simulink model "carTrailerModelDampened"  (R2018b)
settings: Solver=VariableStepAuto  StartTime=0.0  StopTime=StopTime  MaxStep=MaxStep  RelTol=1e-3
InitFcn:
  | SimFramework('model_parameters.json');
model workspace (MAT data in the model file):
  E = 0
  F = 5000
  MaxStep = 0.01
  StopTime = 475
  a1 = 5
  a2 = 2.5
  c = 0
  g = 9.8
  k = 12150
  m1 = 1400
  m2 = 600
  name = 'carTrailerModelDampened'
  u = 0.002
undefined symbols (not defined in the file or in its folder): magnitude
settings Model: Creator=rgeddes  LastModifiedBy=james

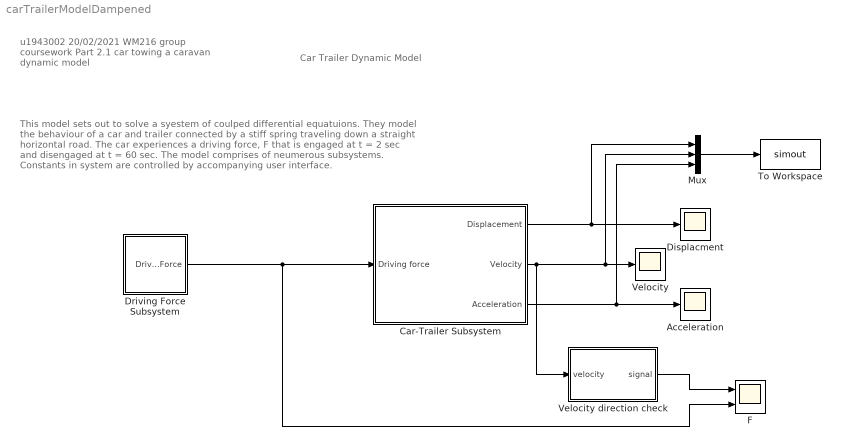
== system carTrailerModelDampened ==
  note: u1943002
      | 20/02/2021
      | WM216 group coursework
      | Part 2.1 car towing a caravan dynamic model
  note: This model sets out to solve a syestem of coulped differential equatuions.
      | They model the behaviour of a car and trailer connected by a stiff spring
      | traveling down a straight horizontal road. The car experiences a driving force, F
      | that is engaged at t = 2 sec and disengaged at t = 60 sec.
      | The model comprises of neumerous subsystems.
      | Constants in system are controlled by accompanying user interface.
  note: Car Trailer Dynamic Model
  Acceleration : Scope
  Car-Trailer Subsystem : Subsystem
      mask help: Combines the behaviour of two ordinary differential equations. Frictional and driving forces can be combined into separate equations for the car and trailer each. The spring force on each body is dependent on the relative displacement between the two bodies. A dampening system was introduced to reduce oscillations.
      mask init:
      | %default values
      | % m1 = 1400;
      | % m2 = 600;
      | % u = 0.002;
      | % a1 = 5;
      | % a2 = 2.5;
      | % g = 9.8;
      | % k = 3*(1800 + 250*9);
      | % c = 0
      | % E = 0
  Displacment : Scope
  Driving Force Subsystem : Subsystem
      mask help: Provindes the driving force F(t) as a function of time.
  F : Scope  NumInputPorts=2
  Mux : Mux  Inputs=3
  To Workspace : ToWorkspace  VariableName=simout  SampleTime=-1
  Velocity : Scope
  Velocity direction check : Subsystem
      mask help: Acts as a way of checking the length of simulation is sufficient. The end of the simulation is determined by visually approximating the point at which the velocity of either the car or trailer becomes negative. This is scaled to the magnitude of driving force, so they are comparable on the same scope.
      mask Help: The time at which peaks on the scoped output  begin reapear after the initial driving force stops can be taken as the time the simulation can be ended.
  wires:
  Car-Trailer Subsystem/3(Acceleration) -> Mux/3, Acceleration/1
  Car-Trailer Subsystem/2(Velocity) -> Velocity direction check/1(velocity), Mux/2, Velocity/1
  Car-Trailer Subsystem/1(Displacement) -> Mux/1, Displacment/1
  Mux/1 -> To Workspace/1
  Velocity direction check/1(signal) -> F/1
  Driving Force Subsystem/1(Driving Force) -> F/2, Car-Trailer Subsystem/1(Driving force)

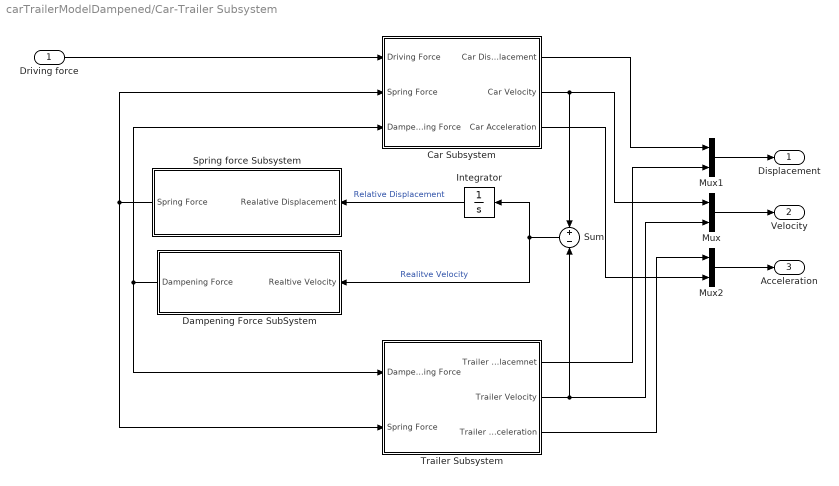
== system carTrailerModelDampened/Car-Trailer Subsystem ==
  Driving force : Inport
  " Car Subsystem" : Subsystem
      mask help:
      | The ODE modeling the behaviour of the car with dampening terms included.
      | x ̈_1=  (F(t))/m_1 -gμx ̇_1-a_1/m_1  〖x ̇_1〗^2-k/m_1  (x_1-x_2 )-c/m_1 (x ̇_1-x ̇_2)
      mask Help:
      | x ̈_1=  (F(t))/m_1 -gμx ̇_1-a_1/m_1  〖x ̇_1〗^2-k/m_1  (x_1-x_2 )-c/m_1 (x ̇_1-x ̇_2)
      | where
      | x _1 is the displacement of the car and its derivatives are given by dot notation.
      | F(t) is the driving force as a function of time.
      | m_1 is the mass of the car.
      | g is acceleration due to gravity.
      | μ is the coefficient of friction.
      | a_1 is the coefficient of air resistance for the car.
      | k is the spring force constant.
      | x_2 is the displacement of the trailer.
      | c is the dampening constant.
  Dampening Force SubSystem : Subsystem
      mask help: As the system undergoes oscilation a dampning sytem was included to explor its effectiveness in reducing oscilations. the dampening force is proportional to the relative velocity between the two bodies. F_d = c (x ̇_1-x ̇_2). the system contains an enable pin to allow the effects of dampening to be turned on and off.
      mask Help:
      | F_d = c (x ̇_1-x ̇_2)
      | where
      | F_d is the dampening force.
      | c is the dampening constant.
      | x ̇_1 is the velocity of the car.
      | x ̇_2 is the velocity of the trailer.
  Integrator : Integrator
  Mux : Mux  Inputs=2
  Mux1 : Mux  Inputs=2
  Mux2 : Mux  Inputs=2
  Spring force Subsystem : Subsystem
      mask help:
      | Spring force is proportional to the length of extension. Extension is given by the difference in displacement between the car and trailer.
      | F_s = k(x_1-x_2)
      mask Help:
      | F_s = k(x_1-x_2)
      | where
      | F_s is the spring force.
      | k is the spring constant.
      | x_1 is the displacement of the car.
      | x_2 is the displacemnet of the trailer.
  Sum : Sum  Inputs=+-
  Trailer Subsystem : Subsystem
      mask help:
      | The ODE modeling the behaviour of the trailer. With dampening terms included.
      | x ̈_2= -gμx ̇_2-a_2/m_2  〖x ̇_1〗^2+k/m_2  (x_1-x_2 )+c/m_2 (x ̇_1-x ̇_2)
      mask Help:
      | x ̈_2= -gμx ̇_2-a_2/m_2  〖x ̇_1〗^2+k/m_2  (x_1-x_2 )+c/m_2 (x ̇_1-x ̇_2)
      | where
      | x _2 is the displacement of the car and its derivatives are given by dot notation.
      | m_2 is the mass of the trailer.
      | g is acceleration due to gravity.
      | μ is the coefficient of friction.
      | a_2 is the coefficient of air resistance for the trailer.
      | k is the spring force constant.
      | x_1 is the displacement of the car.
      | c is the dampening constant.
  Displacement : Outport  VectorParamsAs1DForOutWhenUnconnected=off
  Velocity : Outport  Port=2  VectorParamsAs1DForOutWhenUnconnected=off
  Acceleration : Outport  Port=3  VectorParamsAs1DForOutWhenUnconnected=off
  wires:
  Mux2/1 -> Acceleration/1
  Driving force/1 -> " Car Subsystem"/1(Driving Force)
  Sum/1 -> Dampening Force SubSystem/1(Realtive Velocity), Integrator/1  "Realitve Velocity"
  Spring force Subsystem/1(Spring Force) -> Trailer Subsystem/2(Spring Force), " Car Subsystem"/2(Spring Force)
  Trailer Subsystem/1(Trailer Displacemnet) -> Mux1/2
  " Car Subsystem"/1(Car Displacement) -> Mux1/1
  Trailer Subsystem/3(Trailer Acceleration) -> Mux2/1
  " Car Subsystem"/3(Car Acceleration) -> Mux2/2
  " Car Subsystem"/2(Car Velocity) -> Sum/1, Mux/1
  Trailer Subsystem/2(Trailer Velocity) -> Mux/2, Sum/2
  Mux/1 -> Velocity/1
  Mux1/1 -> Displacement/1
  Integrator/1 -> Spring force Subsystem/1(Realative Displacement)  "Relative Displacement"
  Dampening Force SubSystem/1(Dampening Force) -> " Car Subsystem"/3(Dampening Force), Trailer Subsystem/1(Dampening Force)

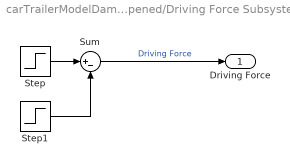
== system carTrailerModelDampened/Driving Force Subsystem ==
  Step : Step  Time=2  After=F  SampleTime=0
  Step1 : Step  Time=60  After=F  SampleTime=0
  Sum : Sum  Inputs=|+-
  Driving Force : Outport  VectorParamsAs1DForOutWhenUnconnected=off
  wires:
  Step/1 -> Sum/1
  Sum/1 -> Driving Force/1  "Driving Force"
  Step1/1 -> Sum/2

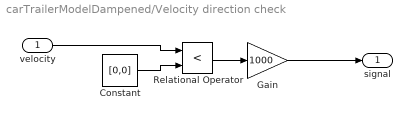
== system carTrailerModelDampened/Velocity direction check ==
  velocity : Inport
  Constant : Constant  Value=[0,0]
  Gain : Gain  Gain=1000
  Relational Operator : RelationalOperator  Operator=<  OutDataTypeStr=boolean  RndMeth=Simplest
  signal : Outport  VectorParamsAs1DForOutWhenUnconnected=off
  wires:
  velocity/1 -> Relational Operator/1
  Relational Operator/1 -> Gain/1
  Constant/1 -> Relational Operator/2
  Gain/1 -> signal/1

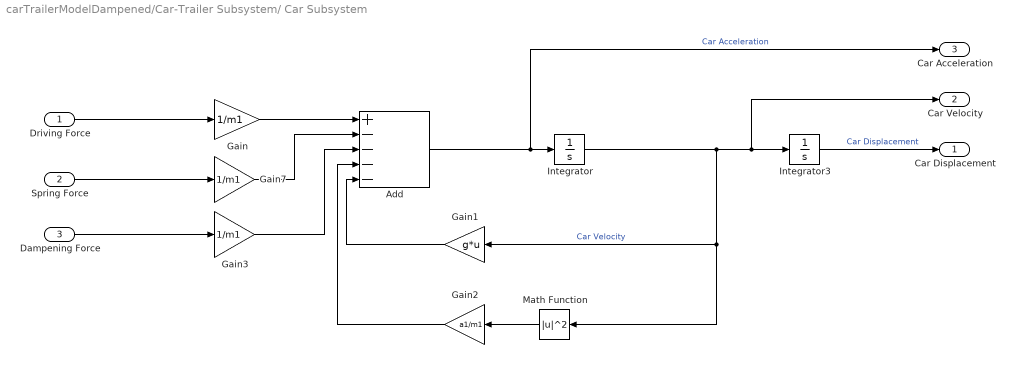
== system carTrailerModelDampened/Car-Trailer Subsystem/ Car Subsystem ==
  Driving Force : Inport
  Spring Force : Inport  Port=2
  Dampening Force : Inport  Port=3
  Add : Sum  Inputs=+----
  Gain : Gain  Gain=1/m1
  Gain1 : Gain  Gain=g*u
  Gain2 : Gain  Gain=a1/m1
  Gain3 : Gain  Gain=1/m1
  Gain7 : Gain  Gain=1/m1
  Integrator : Integrator
  Integrator3 : Integrator
  Math Function : Math  Operator=magnitude^2  SaturateOnIntegerOverflow=on
  Car Displacement : Outport  VectorParamsAs1DForOutWhenUnconnected=off
  Car Velocity : Outport  Port=2  VectorParamsAs1DForOutWhenUnconnected=off
  Car Acceleration : Outport  Port=3  VectorParamsAs1DForOutWhenUnconnected=off
  wires:
  Integrator/1 -> Gain1/1, Math Function/1, Car Velocity/1, Integrator3/1  "Car Velocity"
  Math Function/1 -> Gain2/1
  Gain2/1 -> Add/4
  Gain/1 -> Add/1
  Add/1 -> Car Acceleration/1, Integrator/1  "Car Acceleration"
  Gain1/1 -> Add/5
  Spring Force/1 -> Gain7/1
  Integrator3/1 -> Car Displacement/1  "Car Displacement"
  Driving Force/1 -> Gain/1
  Gain7/1 -> Add/2
  Dampening Force/1 -> Gain3/1
  Gain3/1 -> Add/3

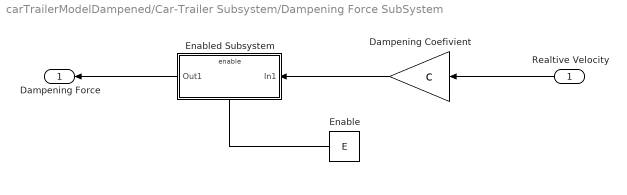
== system carTrailerModelDampened/Car-Trailer Subsystem/Dampening Force SubSystem ==
  Realtive Velocity : Inport
  Dampening Coefivient : Gain  Gain=c
  "Enable " : Constant  Value=E
  Enabled Subsystem : Subsystem  TreatAsAtomicUnit=on
  Dampening Force : Outport  VectorParamsAs1DForOutWhenUnconnected=off
  wires:
  Realtive Velocity/1 -> Dampening Coefivient/1
  Enabled Subsystem/1(Out1) -> Dampening Force/1
  Dampening Coefivient/1 -> Enabled Subsystem/1(In1)
  "Enable "/1 -> Enabled Subsystem/Enable

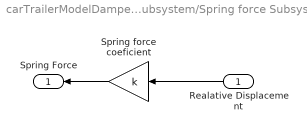
== system carTrailerModelDampened/Car-Trailer Subsystem/Spring force Subsystem ==
  Realative Displacement : Inport
  Spring force coeficient : Gain  Gain=k
  Spring Force : Outport  VectorParamsAs1DForOutWhenUnconnected=off
  wires:
  Realative Displacement/1 -> Spring force coeficient/1
  Spring force coeficient/1 -> Spring Force/1

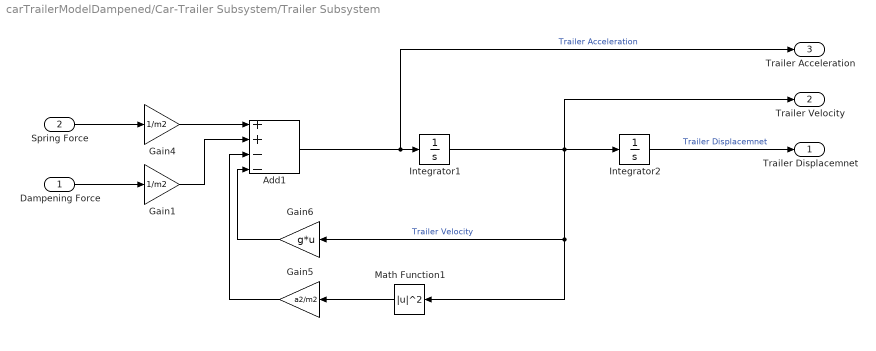
== system carTrailerModelDampened/Car-Trailer Subsystem/Trailer Subsystem ==
  Dampening Force : Inport
  Spring Force : Inport  Port=2
  Add1 : Sum  Inputs=++--
  Gain1 : Gain  Gain=1/m2
  Gain4 : Gain  Gain=1/m2
  Gain5 : Gain  Gain=a2/m2
  Gain6 : Gain  Gain=g*u
  Integrator1 : Integrator
  Integrator2 : Integrator
  Math Function1 : Math  Operator=magnitude^2  SaturateOnIntegerOverflow=on
  Trailer Displacemnet : Outport  VectorParamsAs1DForOutWhenUnconnected=off
  Trailer Velocity : Outport  Port=2  VectorParamsAs1DForOutWhenUnconnected=off
  Trailer Acceleration : Outport  Port=3  VectorParamsAs1DForOutWhenUnconnected=off
  wires:
  Spring Force/1 -> Gain4/1
  Integrator2/1 -> Trailer Displacemnet/1  "Trailer Displacemnet"
  Math Function1/1 -> Gain5/1
  Add1/1 -> Trailer Acceleration/1, Integrator1/1  "Trailer Acceleration"
  Gain5/1 -> Add1/3
  Gain6/1 -> Add1/4
  Integrator1/1 -> Trailer Velocity/1, Integrator2/1, Gain6/1, Math Function1/1  "Trailer Velocity"
  Gain4/1 -> Add1/1
  Dampening Force/1 -> Gain1/1
  Gain1/1 -> Add1/2

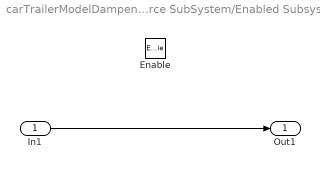
== system carTrailerModelDampened/Car-Trailer Subsystem/Dampening Force SubSystem/Enabled Subsystem ==
  In1 : Inport
  Enable : EnablePort
  Out1 : Outport  VectorParamsAs1DForOutWhenUnconnected=off
  wires:
  In1/1 -> Out1/1
